simulink model "model1"  (R2017a)
settings: Solver=VariableStepAuto  StartTime=0.0  StopTime=20  RelTol=1e-3
values from neighbouring files (symbols this model uses):
  K = 1.098    [param.m]
  taux = 0.977    [param.m]
  Te = 10e-3    (= 0.01)    [param.m]
settings Model: Creator=arek  LastModifiedBy=arek

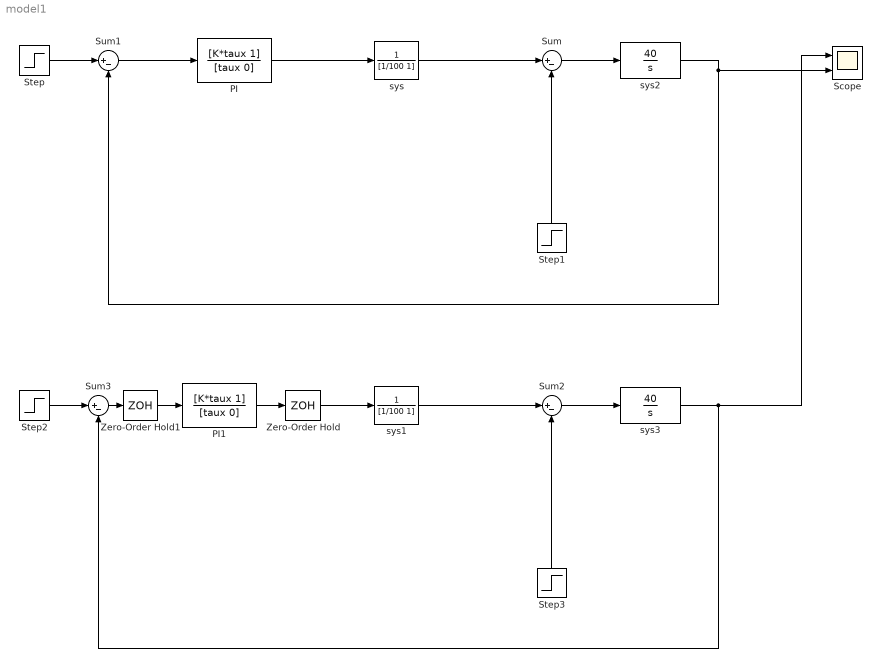
== system model1 ==
  PI : TransferFcn  Numerator=[K*taux 1]  Denominator=[taux 0]
  PI1 : TransferFcn  Numerator=[K*taux 1]  Denominator=[taux 0]
  Scope : Scope  NumInputPorts=2
  Step : Step  SampleTime=0
  Step1 : Step  Time=8  SampleTime=0
  Step2 : Step  SampleTime=0
  Step3 : Step  Time=8  SampleTime=0
  Sum{,1..3} (4 alike) : Sum  Inputs=|+-
  Zero-Order Hold : ZeroOrderHold  SampleTime=Te
  Zero-Order Hold1 : ZeroOrderHold  SampleTime=Te
  sys : TransferFcn  Numerator=1  Denominator=[1/100 1]
  sys1 : TransferFcn  Numerator=1  Denominator=[1/100 1]
  sys2 : TransferFcn  Numerator=40  Denominator=[1 0]
  sys3 : TransferFcn  Numerator=40  Denominator=[1 0]
  wires:
  Sum/1 -> sys2/1
  sys/1 -> Sum/1
  Step1/1 -> Sum/2
  Step/1 -> Sum1/1
  sys2/1 -> Sum1/2, Scope/2
  Sum1/1 -> PI/1
  PI/1 -> sys/1
  Step3/1 -> Sum2/2
  Sum2/1 -> sys3/1
  sys1/1 -> Sum2/1
  sys3/1 -> Sum3/2, Scope/1
  Step2/1 -> Sum3/1
  Zero-Order Hold/1 -> sys1/1
  PI1/1 -> Zero-Order Hold/1
  Sum3/1 -> Zero-Order Hold1/1
  Zero-Order Hold1/1 -> PI1/1
